simulink library "EdgeCounter"  (R2018b)
settings: Solver=VariableStepAuto  StartTime=0.0  StopTime=10.0  RelTol=1e-3
libraries: simulink x2
settings Model: Creator=moritahiromitsu  LastModifiedBy=moritahiromitsu

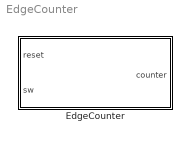
== system EdgeCounter ==
  EdgeCounter : Subsystem  TreatAsAtomicUnit=on

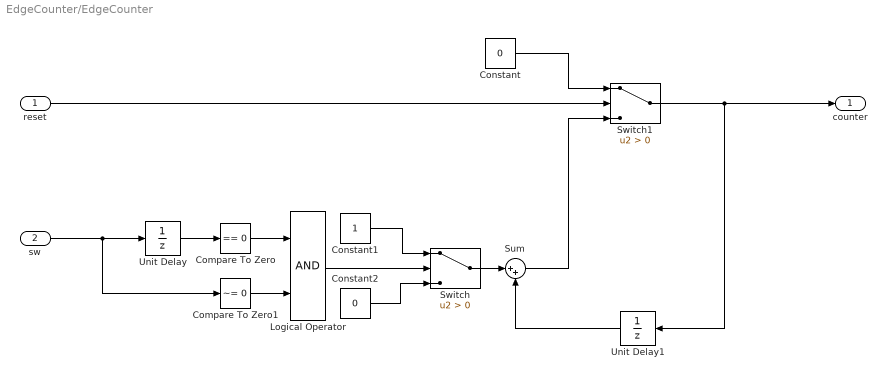
== system EdgeCounter/EdgeCounter ==
  reset : Inport
  sw : Inport  Port=2
  Compare To Zero : simulink/Logic and Bit Operations/Compare To Zero  relop===  OutDataTypeStr=boolean
  Compare To Zero1 : simulink/Logic and Bit Operations/Compare To Zero  relop=~=  OutDataTypeStr=boolean
  Constant : Constant  Value=0
  Constant1 : Constant  OutDataTypeStr=uint8
  Constant2 : Constant  Value=0  OutDataTypeStr=uint8
  Logical Operator : Logic  AllPortsSameDT=off  OutDataTypeStr=boolean
  Sum : Sum  Inputs=|++  RndMeth=Zero  SaturateOnIntegerOverflow=on
  Switch : Switch  Criteria=u2 > Threshold  OutDataTypeStr=uint8  RndMeth=Zero  SaturateOnIntegerOverflow=on
  Switch1 : Switch  Criteria=u2 > Threshold  OutDataTypeStr=uint8  RndMeth=Zero  SaturateOnIntegerOverflow=on
  Unit Delay : UnitDelay  SampleTime=-1
  Unit Delay1 : UnitDelay  SampleTime=-1
  counter : Outport
  wires:
  Unit Delay/1 -> Compare To Zero/1
  sw/1 -> Compare To Zero1/1, Unit Delay/1
  Compare To Zero/1 -> Logical Operator/1
  Compare To Zero1/1 -> Logical Operator/2
  Switch/1 -> Sum/1
  reset/1 -> Switch1/2
  Sum/1 -> Switch1/3
  Switch1/1 -> Unit Delay1/1, counter/1
  Unit Delay1/1 -> Sum/2
  Constant/1 -> Switch1/1
  Constant1/1 -> Switch/1
  Logical Operator/1 -> Switch/2
  Constant2/1 -> Switch/3
